simulink model "c250_bb2"  (R2012b)
settings: Solver=VariableStepDiscrete  SolverMode=SingleTasking  StartTime=0.0  StopTime=10000  RelTol=1e-3
libraries: xbsIndex_r4 x4529, casper_library_misc x63, xps_library x6
(part 3 of 39)

== system c250_bb2/BufferedSwitch ==
  fft_data : Inport
  data_rdy : Inport  Port=2
  fft_bin0 : Inport  Port=3
  fft_bin1 : Inport  Port=4
  fft_bin2 : Inport  Port=5
  fft_bin3 : Inport  Port=6
  ch_in : Inport  Port=7
  Adress Counter1 : xbsIndex_r4/Counter  cnt_type=Free Running  cnt_to=Inf  operation=Up  start_count=0  cnt_by_val=1  arith_type=Unsigned  n_bits=8  bin_pt=0  load_pin=off  rst=on  en=on  explicit_period=on  period=1  dbl_ovrd=off  use_behavioral_HDL=off  implementation=Fabric  use_rpm=off  block_type=counter
  Adress Counter2 : xbsIndex_r4/Counter  cnt_type=Free Running  cnt_to=Inf  operation=Up  start_count=0  cnt_by_val=1  arith_type=Unsigned  n_bits=8  bin_pt=0  load_pin=off  rst=on  en=on  explicit_period=on  period=1  dbl_ovrd=off  use_behavioral_HDL=off  implementation=Fabric  use_rpm=off  block_type=counter
  Convert1 : xbsIndex_r4/Convert  gui_display_data_type=Boolean  arith_type=Boolean  n_bits=16  bin_pt=13  float_type=Single  exp_bits=8  fraction_bits=24  quantization=Truncate  overflow=Wrap  en=off  latency=0  dbl_ovrd=off  pipeline=off  block_type=convert
      settings: block_version=11.4
  Inverter4 : xbsIndex_r4/Inverter  en=off  latency=0  dbl_ovrd=off  block_type=inv
  Mux{1..12} (12 alike) : xbsIndex_r4/Mux  inputs=2  en=off  latency=1  precision=Full  arith_type=Unsigned  n_bits=16  bin_pt=14  quantization=Truncate  overflow=Wrap  dbl_ovrd=off  block_type=mux
  Slice{1..7,12} (8 alike) : xbsIndex_r4/Slice  nbits=8  boolean_output=off  mode=Lower Bit Location + Width  bit1=0  base1=MSB of Input  bit0=3  base0=LSB of Input  dbl_ovrd=off  block_type=slice
      settings: block_version=10.1.3
  Slice{8..11} (4 alike) : xbsIndex_r4/Slice  nbits=3  boolean_output=off  mode=Lower Bit Location + Width  bit1=0  base1=MSB of Input  bit0=0  base0=LSB of Input  dbl_ovrd=off  block_type=slice
      settings: block_version=10.1.3
  ram_buff : Subsystem
  ram_buff1 : Subsystem
  ram_buff2 : Subsystem
  ram_buff3 : Subsystem
  ram_buff4 : Subsystem
  ram_buff5 : Subsystem
  ram_buff6 : Subsystem
  ram_buff7 : Subsystem
  selector : xbsIndex_r4/Counter  cnt_type=Free Running  cnt_to=Inf  operation=Up  start_count=0  cnt_by_val=1  arith_type=Unsigned  n_bits=1  bin_pt=0  load_pin=off  rst=off  en=on  explicit_period=on  period=1  dbl_ovrd=off  use_behavioral_HDL=off  implementation=Fabric  use_rpm=off  block_type=counter
  data_rdy_out : Outport
  data_out0 : Outport  Port=2
  data_out1 : Outport  Port=3
  data_out2 : Outport  Port=4
  data_out3 : Outport  Port=5
  ch_out : Outport  Port=6
  wires:
  data_rdy/1 -> data_rdy_out/1, Adress Counter1/1, Adress Counter2/1, selector/1
  fft_data/1 -> ram_buff1/3(data_in), ram_buff2/3(data_in), ram_buff3/3(data_in), ram_buff4/3(data_in), ram_buff5/3(data_in), ram_buff6/3(data_in), ram_buff7/3(data_in), ram_buff/3(data_in)
  selector/1 -> Convert1/1
  Inverter4/1 -> Mux8/1, Mux9/1, Mux7/1, Adress Counter1/2, Mux3/1, ram_buff4/4(we), ram_buff7/4(we), ram_buff6/4(we), ram_buff5/4(we)
  fft_bin0/1 -> Slice4/1, Slice1/1, Slice9/1
  fft_bin1/1 -> Slice5/1, Slice2/1, Slice8/1
  fft_bin2/1 -> Slice10/1, Slice6/1, Slice3/1
  fft_bin3/1 -> Slice11/1, Slice7/1, Slice12/1
  Mux1/1 -> ram_buff/2(addr)
  Mux4/1 -> ram_buff1/2(addr)
  Mux5/1 -> ram_buff2/2(addr)
  Mux6/1 -> ram_buff3/2(addr)
  Mux3/1 -> ram_buff4/2(addr)
  Mux7/1 -> ram_buff5/2(addr)
  Mux8/1 -> ram_buff6/2(addr)
  Mux9/1 -> ram_buff7/2(addr)
  Adress Counter2/1 -> Mux1/3, Mux4/3, Mux5/3, Mux6/3
  Adress Counter1/1 -> Mux7/3, Mux8/3, Mux9/3, Mux3/3
  Mux2/1 -> data_out0/1
  ch_in/1 -> ch_out/1
  Slice1/1 -> Mux1/2
  Slice2/1 -> Mux4/2
  Slice3/1 -> Mux5/2
  Slice4/1 -> Mux3/2
  Slice5/1 -> Mux7/2
  Slice6/1 -> Mux8/2
  Slice7/1 -> Mux9/2
  Slice11/1 -> ram_buff7/1(addr_pre), ram_buff3/1(addr_pre)
  Slice10/1 -> ram_buff6/1(addr_pre), ram_buff2/1(addr_pre)
  Slice8/1 -> ram_buff5/1(addr_pre), ram_buff1/1(addr_pre)
  Slice9/1 -> ram_buff/1(addr_pre), ram_buff4/1(addr_pre)
  Convert1/1 -> ram_buff3/4(we), ram_buff2/4(we), ram_buff1/4(we), ram_buff/4(we), Mux12/1, Mux11/1, Mux10/1, Mux2/1, Mux5/1, Mux6/1, Inverter4/1, Mux4/1, Adress Counter2/2, Mux1/1
  Slice12/1 -> Mux6/2
  ram_buff/1(data_out) -> Mux2/2
  ram_buff4/1(data_out) -> Mux2/3
  ram_buff1/1(data_out) -> Mux10/2
  ram_buff2/1(data_out) -> Mux11/2
  ram_buff3/1(data_out) -> Mux12/2
  ram_buff5/1(data_out) -> Mux10/3
  ram_buff6/1(data_out) -> Mux11/3
  ram_buff7/1(data_out) -> Mux12/3
  Mux10/1 -> data_out1/1
  Mux11/1 -> data_out2/1
  Mux12/1 -> data_out3/1
